simulink model "Observador_ex1_2015a"  (Simulink 8.5)
settings: Solver=ode45  SolverMode=SingleTasking  StartTime=0.0  StopTime=5  RelTol=1e-3
values from neighbouring files (symbols this model uses):
  A = [1 -1 0.01 0.12]    [Real_Esta_Disc_Ref.m]    (also in Routh_Hurwitz.m = [0 1 0;0 0 1;-160 -56 -14]; Smulacro_Parcial_Final.m = matrizA; observador_estados_ex1.m = [-20 1 ;-1 0]; tercer_orden.m = 1)
  b = [5 1 2]    [Realimentacion_Acker.m]    (also in Resumen_PrimerCorte_obsContrRouth.m = [1]; RouthPrueba.m = [rand(1,((l-1)/2)),0]; observador_estados_ex1.m = [1; 0])
  c = zeros(l,l1)    [RouthPrueba.m]    (also in observador_estados_ex1.m = [0 1])
  l = length(e)    [RouthPrueba.m]    (also in observador_estados_ex1.m = k')
settings Model: Creator=Sergio  LastModifiedBy=Sergio  CovMetricSettings=dwe  CovHtmlReporting=off  covSaveCumulativeToWorkspaceVar=off  CovSaveSingleToWorkspaceVar=off  CovExternalEMLEnable=on
settings DataIOCC: LimitDataPoints=off  SaveFormat=Dataset  SignalLoggingSaveFormat=Dataset  ReturnWorkspaceOutputs=on
settings OptimizationCC: ExpressionDepthLimit=128
settings DebuggingCC: UnderspecifiedInitializationDetection=Simplified  MergeDetectMultiDrivingBlocksExec=error  FcnCallInpInsideContextMsg=EnableAllAsError  StateNameClashWarn=none  SFUnexpectedBacktrackingDiag=error  SFNoUnconditionalDefaultTransitionDiag=error
settings HardwareCC: ProdBitPerPointer=64  ProdLargestAtomicFloat=Float  ProdIntDivRoundTo=Zero  ProdEndianess=LittleEndian  ProdHWDeviceType=Specified
settings ModelReferenceCC: PropagateSignalLabelsOutOfModel=on
settings SFSimCC: SimUseLocalCustomCode=on
settings RTWCC: RTWUseLocalCustomCode=on
settings GRTTargetCC: TargetLangStandard=C99 (ISO)  CombineOutputUpdateFcns=on  GRTInterface=off

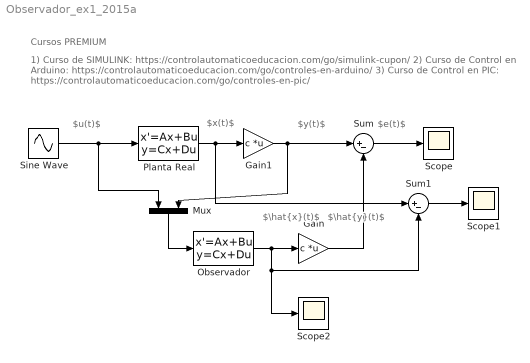
== system Observador_ex1_2015a ==
  note: Cursos PREMIUM
  note: 1) Curso de SIMULINK: https://controlautomaticoeducacion.com/go/simulink-cupon/
      | 2) Curso de Control en Arduino: https://controlautomaticoeducacion.com/go/controles-en-arduino/
      | 3) Curso de Control en PIC: https://controlautomaticoeducacion.com/go/controles-en-pic/
  note: $\hat{y}(t)$
  note: $y(t)$
  note: $u(t)$
  note: $e(t)$
  note: $\hat{x}(t)$
  note: $x(t)$
  Gain : Gain  Gain=c  Multiplication=Matrix(K*u)
  Gain1 : Gain  Gain=c  Multiplication=Matrix(K*u)
  Mux : Mux  Inputs=2
  Observador : StateSpace  A=A-l*c  B=[b,l]  C=eye(2)  D=zeros(2)  X0=[0; 0]
  Planta Real : StateSpace  A=A  B=b  C=eye(2)  D=[0 0]'  X0=[1 0]
  Scope : Scope
      settings: TimeRange=auto  MaxDataPoints=5000  SaveToWorkspace=off  SaveName=ScopeData  YMin=-0.22372  YMax=1.13597  SampleTime=-1
  Scope1 : Scope
      settings: TimeRange=auto  MaxDataPoints=5000  SaveToWorkspace=off  YMin=-0.84808  YMax=1.20534  SampleTime=-1
  Scope2 : Scope
      settings: TimeRange=auto  MaxDataPoints=5000  SaveToWorkspace=off  SaveName=ScopeData2  YMin=-26.69092  YMax=233.65466  SampleTime=-1
  Sine Wave : Sin  Frequency=0.5  SampleTime=0
  Sum : Sum  Inputs=|+-
  Sum1 : Sum  Inputs=|+-
  wires:
  Mux/1 -> Observador/1
  Planta Real/1 -> Sum1/1, Gain1/1
  Sine Wave/1 -> Mux/1, Planta Real/1
  Observador/1 -> Scope2/1, Sum1/2, Gain/1
  Gain/1 -> Sum/2
  Sum/1 -> Scope/1
  Gain1/1 -> Mux/2, Sum/1
  Sum1/1 -> Scope1/1
